simulink model "Modello_Irb1300_R2022a_ultima"  (R2022a)
settings: Solver=VariableStepAuto  StartTime=0.0  StopTime=37  RelTol=1e-3
undefined symbols (not defined in the file or in its folder): DiscIntNeverNeededParam
libraries: vrlib x3, simulink x1
settings Model: Creator=giaki  LastModifiedBy=adewa
settings ModelReferenceCC: EnableRefExpFcnMdlSchedulingChecks=off
settings RTWCC: Description=Generic Real-Time Target  GPUComputeCapability=5.0

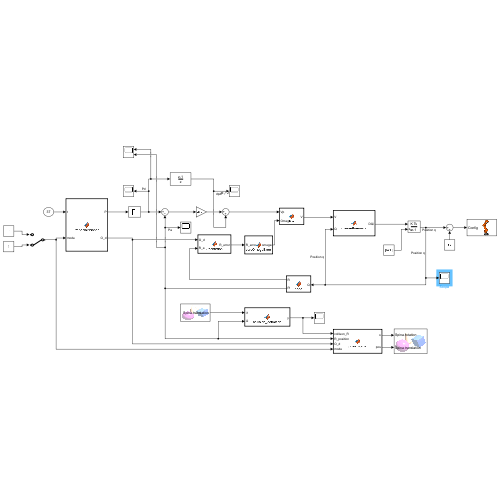
[thumbnail: Simulink's stored preview of the top-level diagram]
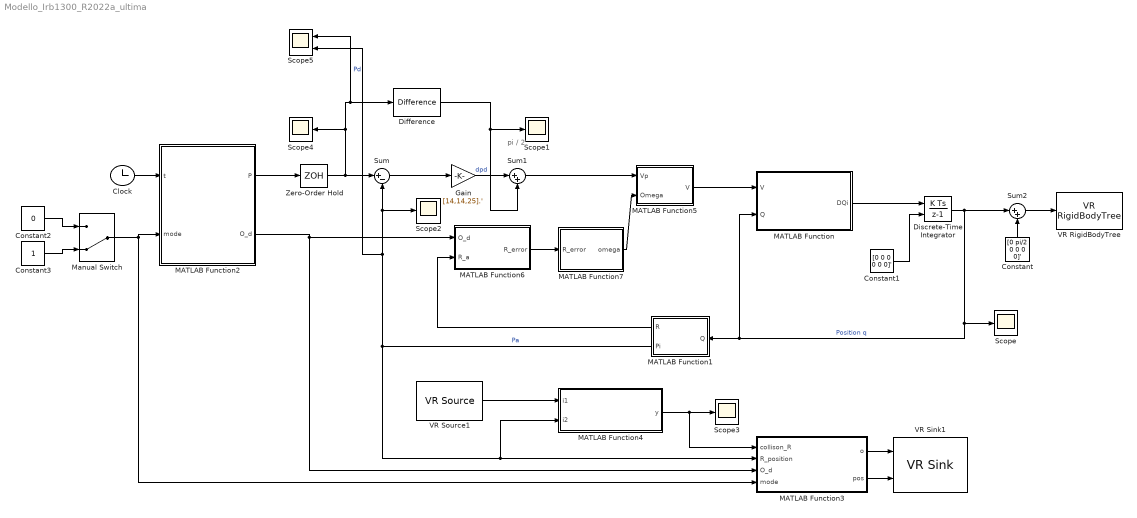
== system Modello_Irb1300_R2022a_ultima ==
  note: pi / 2
  Clock : Clock
  Constant : Constant  Value=[0 pi/2 0 0 0 0]'
  Constant1 : Constant  Value=[0 0 0 0 0 0]'
  Constant2 : Constant  Value=0
  Constant3 : Constant
  Difference : simulink/Discrete/Difference  ICPrevInput=[0.66, 0, 1.015].'  OutMin=[]  OutMax=[]  OutDataType=fixdt(1, 16)  OutScaling=2^-10  DoSatur=off
  Discrete-Time Integrator : DiscreteIntegrator  InitialConditionSource=external  SampleTime=-1  OutMin=[2]  ICPrevOutput=DiscIntNeverNeededParam  ICPrevScaledInput=DiscIntNeverNeededParam
  Gain : Gain  Gain=[14,14,25].'
  MATLAB Function : MATLAB Function  TreatAsAtomicUnit=on
  MATLAB Function1 : MATLAB Function  TreatAsAtomicUnit=on
  MATLAB Function2 : MATLAB Function  TreatAsAtomicUnit=on
  MATLAB Function3 : MATLAB Function  TreatAsAtomicUnit=on
  MATLAB Function4 : MATLAB Function  TreatAsAtomicUnit=on
  MATLAB Function5 : MATLAB Function  TreatAsAtomicUnit=on
  MATLAB Function6 : MATLAB Function  TreatAsAtomicUnit=on
  MATLAB Function7 : MATLAB Function  TreatAsAtomicUnit=on
  Manual Switch : ManualSwitch  CurrentSetting=0
  Scope{,1..4} (5 alike) : Scope
  Scope5 : Scope  NumInputPorts=2
  Sum : Sum  Inputs=|+-
  Sum1 : Sum  Inputs=|++
  Sum2 : Sum  Inputs=|++
  VR RigidBodyTree : vrlib/VR RigidBodyTree  VrmlFile=robot_scene_2.x3d  RBT=Irb1300  useRBT=on  Ts=0.1  ForceViewerOpen=on
      settings: SourceProductBaseCode=SL
  VR Sink1 : vrlib/VR Sink  InstantiateOnLoad=on  SampleTime=0.1  ViewEnable=on  RemoteChange=off  RemoteView=off  FieldsWritten=Spina.rotation.4.1.1.double#Spina.translation.3.1.1.double  WorldFileName=robot_scene_2.x3d  WorldDescription=Simple Robot Scene  AutoView=off  VideoDimensions=[]  AllowVariableSize=off
  VR Source1 : vrlib/VR Source  InstantiateOnLoad=on  SampleTime=0.1  ViewEnable=on  RemoteChange=off  RemoteView=off  FieldsRead=Spina.translation.1.3.1.double  WorldFileName=robot_scene_2.x3d  WorldDescription=Simple Robot Scene  AutoView=off  VideoDimensions=[]  AllowVariableSize=off
      settings: SourceProductBaseCode=SL
  Zero-Order Hold : ZeroOrderHold  SampleTime=0.05
  wires:
  Discrete-Time Integrator/1 -> Sum2/1, Scope/1, MATLAB Function/2(Q), MATLAB Function1/1(Q)  "Position q"
  Constant/1 -> Sum2/2
  Constant1/1 -> Discrete-Time Integrator/2
  Sum2/1 -> VR RigidBodyTree/1
  Difference/1 -> Scope1/1, Sum1/2  "dpd"
  Clock/1 -> MATLAB Function2/1(t)
  MATLAB Function/1(DQi) -> Discrete-Time Integrator/1
  Gain/1 -> Sum1/1
  MATLAB Function4/1(y) -> MATLAB Function3/1(collison_R), Scope3/1
  VR Source1/1 -> MATLAB Function4/1(i1)
  MATLAB Function2/1(P) -> Zero-Order Hold/1
  MATLAB Function3/2(pos) -> VR Sink1/2
  Zero-Order Hold/1 -> Scope4/1, Scope5/1, Difference/1, Sum/1  "Pd"
  Sum/1 -> Gain/1
  MATLAB Function1/1(R) -> MATLAB Function6/2(R_a)
  Sum1/1 -> MATLAB Function5/1(Vp)
  MATLAB Function5/1(V) -> MATLAB Function/1(V)
  MATLAB Function6/1(R_error) -> MATLAB Function7/1(R_error)
  MATLAB Function7/1(omega) -> MATLAB Function5/2(Omega)
  MATLAB Function1/2(Pi) -> Scope5/2, Sum/2, Scope2/1, MATLAB Function4/2(i2), MATLAB Function3/2(R_position)  "Pa"
  MATLAB Function2/2(O_d) -> MATLAB Function6/1(O_d), MATLAB Function3/3(O_d)
  MATLAB Function3/1(o) -> VR Sink1/1
  Manual Switch/1 -> MATLAB Function3/4(mode), MATLAB Function2/2(mode)
  Constant2/1 -> Manual Switch/1
  Constant3/1 -> Manual Switch/2

== matlab function Modello_Irb1300_R2022a_ultima/MATLAB Function1 ==
  data: R output; Q input; Pi output
function [R,Pi] = posa(Q)

th1 = Q(1);
th2 = Q(2);
th3 = Q(3);
th4 = Q(4);
th5 = Q(5);
th6 = Q(6);

% Matrice di trasformazione 4x4 calcolata nella posizione Q
T = [
    [sin(th6)*(cos(th4)*sin(th1) + sin(th4)*(cos(th1)*sin(th3)*sin(th2 + pi/2) - cos(th1)*cos(th3)*cos(th2 + pi/2))) + cos(th6)*(cos(th5)*(sin(th1)*sin(th4) - cos(th4)*(cos(th1)*sin(th3)*sin(th2 + pi/2) - cos(th1)*cos(th3)*cos(th2 + pi/2))) - sin(th5)*(cos(th1)*cos(th3)*sin(th2 + pi/2) + cos(th1)*cos(th2 + pi/2)*sin(th3))), cos(th6)*(cos(th4)*sin(th1) + sin(th4)*(cos(th1)*sin(th3)*sin(th2 + pi/2) - cos(th1)*cos(th3)*cos(th2 + pi/2))) - sin(th6)*(cos(th5)*(sin(th1)*sin(th4) - cos(th4)*(cos(th1)*sin(th3)*sin(th2 + pi/2) - cos(th1)*cos(th3)*cos(th2 + pi/2))) - sin(th5)*(cos(th1)*cos(th3)*sin(th2 + pi/2) + cos(th1)*cos(th2 + pi/2)*sin(th3))), sin(th5)*(sin(th1)*sin(th4) - cos(th4)*(cos(th1)*sin(th3)*sin(th2 + pi/2) - cos(th1)*cos(th3)*cos(th2 + pi/2))) + cos(th5)*(cos(th1)*cos(th3)*sin(th2 + pi/2) + cos(th1)*cos(th2 + pi/2)*sin(th3)), cos(th1)/20 + (17*cos(th1)*cos(th2 + pi/2))/40 + (9*sin(th5)*(sin(th1)*sin(th4) - cos(th4)*(cos(th1)*sin(th3)*sin(th2 + pi/2) - cos(th1)*cos(th3)*cos(th2 + pi/2))))/50 + (9*cos(th5)*(cos(th1)*cos(th3)*sin(th2 + pi/2) + cos(th1)*cos(th2 + pi/2)*sin(th3)))/50 + (17*cos(th1)*cos(th3)*sin(th2 + pi/2))/40 + (17*cos(th1)*cos(th2 + pi/2)*sin(th3))/40 - (cos(th1)*sin(th3)*sin(th2 + pi/2))/25 + (cos(th1)*cos(th3)*cos(th2 + pi/2))/25]
    [-sin(th6)*(cos(th1)*cos(th4) + sin(th4)*(cos(th3)*cos(th2 + pi/2)*sin(th1) - sin(th1)*sin(th3)*sin(th2 + pi/2))) - cos(th6)*(cos(th5)*(cos(th1)*sin(th4) - cos(th4)*(cos(th3)*cos(th2 + pi/2)*sin(th1) - sin(th1)*sin(th3)*sin(th2 + pi/2))) + sin(th5)*(cos(th3)*sin(th1)*sin(th2 + pi/2) + cos(th2 + pi/2)*sin(th1)*sin(th3))), sin(th6)*(cos(th5)*(cos(th1)*sin(th4) - cos(th4)*(cos(th3)*cos(th2 + pi/2)*sin(th1) - sin(th1)*sin(th3)*sin(th2 + pi/2))) + sin(th5)*(cos(th3)*sin(th1)*sin(th2 + pi/2) + cos(th2 + pi/2)*sin(th1)*sin(th3))) - cos(th6)*(cos(th1)*cos(th4) + sin(th4)*(cos(th3)*cos(th2 + pi/2)*sin(th1) - sin(th1)*sin(th3)*sin(th2 + pi/2))), cos(th5)*(cos(th3)*sin(th1)*sin(th2 + pi/2) + cos(th2 + pi/2)*sin(th1)*sin(th3)) - sin(th5)*(cos(th1)*sin(th4) - cos(th4)*(cos(th3)*cos(th2 + pi/2)*sin(th1) - sin(th1)*sin(th3)*sin(th2 + pi/2))), sin(th1)/20 + (17*cos(th2 + pi/2)*sin(th1))/40 - (9*sin(th5)*(cos(th1)*sin(th4) - cos(th4)*(cos(th3)*cos(th2 + pi/2)*sin(th1) - sin(th1)*sin(th3)*sin(th2 + pi/2))))/50 + (9*cos(th5)*(cos(th3)*sin(th1)*sin(th2 + pi/2) + cos(th2 + pi/2)*sin(th1)*sin(th3)))/50 + (cos(th3)*cos(th2 + pi/2)*sin(th1))/25 + (17*cos(th3)*sin(th1)*sin(th2 + pi/2))/40 + (17*cos(th2 + pi/2)*sin(th1)*sin(th3))/40 - (sin(th1)*sin(th3)*sin(th2 + pi/2))/25]
    [cos(th6)*(sin(th5)*(cos(th3)*cos(th2 + pi/2) - sin(th3)*sin(th2 + pi/2)) + cos(th4)*cos(th5)*(cos(th3)*sin(th2 + pi/2) + cos(th2 + pi/2)*sin(th3))) - sin(th4)*sin(th6)*(cos(th3)*sin(th2 + pi/2) + cos(th2 + pi/2)*sin(th3)), -sin(th6)*(sin(th5)*(cos(th3)*cos(th2 + pi/2) - sin(th3)*sin(th2 + pi/2)) + cos(th4)*cos(th5)*(cos(th3)*sin(th2 + pi/2) + cos(th2 + pi/2)*sin(th3))) - cos(th6)*sin(th4)*(cos(th3)*sin(th2 + pi/2) + cos(th2 + pi/2)*sin(th3)), cos(th4)*sin(th5)*(cos(th3)*sin(th2 + pi/2) + cos(th2 + pi/2)*sin(th3)) - cos(th5)*(cos(th3)*cos(th2 + pi/2) - sin(th3)*sin(th2 + pi/2)), (17*sin(th2 + pi/2))/40 - (17*cos(th3)*cos(th2 + pi/2))/40 + (cos(th3)*sin(th2 + pi/2))/25 + (cos(th2 + pi/2)*sin(th3))/25 + (17*sin(th3)*sin(th2 + pi/2))/40 - (9*cos(th5)*(cos(th3)*cos(th2 + pi/2) - sin(th3)*sin(th2 + pi/2)))/50 + (9*cos(th4)*sin(th5)*(cos(th3)*sin(th2 + pi/2) + cos(th2 + pi/2)*sin(th3)))/50 + 68/125]
    [0, 0, 0, 1]
];

% Estrai la posizione (3x1)
Pi_position = T(1:3, 4);

% Estrai la matrice di rotazione (3x3)
R = T(1:3, 1:3);


% Restituisci la posizione
Pi = [Pi_position];
end

== matlab function Modello_Irb1300_R2022a_ultima/MATLAB Function ==
  data: V input; DQi output; Q input
function DQi = inverseKinematic(V,Q)

th1 = Q(1);
th2 = Q(2);
th3 = Q(3);
th4 = Q(4);
th5 = Q(5);
th6 = Q(6);


% cosiderando sia le traslazioni che le orientazioni viene utilizzato il seguente J che si riferisce al jacobiano completo J = Jp + Jo 
J = [
[(9*sin(th5)*(cos(th1)*sin(th4) - cos(th4)*(cos(th3)*cos(th2 + pi/2)*sin(th1) - sin(th1)*sin(th3)*sin(th2 + pi/2))))/50 - (17*cos(th2 + pi/2)*sin(th1))/40 - sin(th1)/20 - (9*cos(th5)*(cos(th3)*sin(th1)*sin(th2 + pi/2) + cos(th2 + pi/2)*sin(th1)*sin(th3)))/50 - (cos(th3)*cos(th2 + pi/2)*sin(th1))/25 - (17*cos(th3)*sin(th1)*sin(th2 + pi/2))/40 - (17*cos(th2 + pi/2)*sin(th1)*sin(th3))/40 + (sin(th1)*sin(th3)*sin(th2 + pi/2))/25, (17*cos(th1)*cos(th3)*cos(th2 + pi/2))/40 - (9*cos(th5)*(cos(th1)*sin(th3)*sin(th2 + pi/2) - cos(th1)*cos(th3)*cos(th2 + pi/2)))/50 - (cos(th1)*cos(th3)*sin(th2 + pi/2))/25 - (cos(th1)*cos(th2 + pi/2)*sin(th3))/25 - (17*cos(th1)*sin(th3)*sin(th2 + pi/2))/40 - (9*cos(th4)*sin(th5)*(cos(th1)*cos(th3)*sin(th2 + pi/2) + cos(th1)*cos(th2 + pi/2)*sin(th3)))/50 - (17*cos(th1)*sin(th2 + pi/2))/40, (17*cos(th1)*cos(th3)*cos(th2 + pi/2))/40 - (cos(th1)*cos(th3)*sin(th2 + pi/2))/25 - (cos(th1)*cos(th2 + pi/2)*sin(th3))/25 - (17*cos(th1)*sin(th3)*sin(th2 + pi/2))/40 - (9*cos(th4)*sin(th5)*(cos(th1)*cos(th3)*sin(th2 + pi/2) + cos(th1)*cos(th2 + pi/2)*sin(th3)))/50 - (9*cos(th5)*(cos(th1)*sin(th3)*sin(th2 + pi/2) - cos(th1)*cos(th3)*cos(th2 + pi/2)))/50,  (9*sin(th5)*(cos(th4)*sin(th1) + sin(th4)*(cos(th1)*sin(th3)*sin(th2 + pi/2) - cos(th1)*cos(th3)*cos(th2 + pi/2))))/50,   (9*cos(th5)*(sin(th1)*sin(th4) - cos(th4)*(cos(th1)*sin(th3)*sin(th2 + pi/2) - cos(th1)*cos(th3)*cos(th2 + pi/2))))/50 - (9*sin(th5)*(cos(th1)*cos(th3)*sin(th2 + pi/2) + cos(th1)*cos(th2 + pi/2)*sin(th3)))/50,                                                                                                                                                                                                  0]
[cos(th1)/20 + (17*cos(th1)*cos(th2 + pi/2))/40 + (9*sin(th5)*(sin(th1)*sin(th4) - cos(th4)*(cos(th1)*sin(th3)*sin(th2 + pi/2) - cos(th1)*cos(th3)*cos(th2 + pi/2))))/50 + (9*cos(th5)*(cos(th1)*cos(th3)*sin(th2 + pi/2) + cos(th1)*cos(th2 + pi/2)*sin(th3)))/50 + (17*cos(th1)*cos(th3)*sin(th2 + pi/2))/40 + (17*cos(th1)*cos(th2 + pi/2)*sin(th3))/40 - (cos(th1)*sin(th3)*sin(th2 + pi/2))/25 + (cos(th1)*cos(th3)*cos(th2 + pi/2))/25, (9*cos(th5)*(cos(th3)*cos(th2 + pi/2)*sin(th1) - sin(th1)*sin(th3)*sin(th2 + pi/2)))/50 - (17*sin(th1)*sin(th2 + pi/2))/40 + (17*cos(th3)*cos(th2 + pi/2)*sin(th1))/40 - (cos(th3)*sin(th1)*sin(th2 + pi/2))/25 - (cos(th2 + pi/2)*sin(th1)*sin(th3))/25 - (17*sin(th1)*sin(th3)*sin(th2 + pi/2))/40 - (9*cos(th4)*sin(th5)*(cos(th3)*sin(th1)*sin(th2 + pi/2) + cos(th2 + pi/2)*sin(th1)*sin(th3)))/50, (9*cos(th5)*(cos(th3)*cos(th2 + pi/2)*sin(th1) - sin(th1)*sin(th3)*sin(th2 + pi/2)))/50 + (17*cos(th3)*cos(th2 + pi/2)*sin(th1))/40 - (cos(th3)*sin(th1)*sin(th2 + pi/2))/25 - (cos(th2 + pi/2)*sin(th1)*sin(th3))/25 - (17*sin(th1)*sin(th3)*sin(th2 + pi/2))/40 - (9*cos(th4)*sin(th5)*(cos(th3)*sin(th1)*sin(th2 + pi/2) + cos(th2 + pi/2)*sin(th1)*sin(th3)))/50, -(9*sin(th5)*(cos(th1)*cos(th4) + sin(th4)*(cos(th3)*cos(th2 + pi/2)*sin(th1) - sin(th1)*sin(th3)*sin(th2 + pi/2))))/50, - (9*cos(th5)*(cos(th1)*sin(th4) - cos(th4)*(cos(th3)*cos(th2 + pi/2)*sin(th1) - sin(th1)*sin(th3)*sin(th2 + pi/2))))/50 - (9*sin(th5)*(cos(th3)*sin(th1)*sin(th2 + pi/2) + cos(th2 + pi/2)*sin(th1)*sin(th3)))/50,                                                                                                                                                                                                  0]
[                                                                                                                                                                                                                                                                                                                                                                                                                                          0,                                                                                  (17*cos(th2 + pi/2))/40 + (cos(th3)*cos(th2 + pi/2))/25 + (17*cos(th3)*sin(th2 + pi/2))/40 + (17*cos(th2 + pi/2)*sin(th3))/40 - (sin(th3)*sin(th2 + pi/2))/25 + (9*cos(th5)*(cos(th3)*sin(th2 + pi/2) + cos(th2 + pi/2)*sin(th3)))/50 + (9*cos(th4)*sin(th5)*(cos(th3)*cos(th2 + pi/2) - sin(th3)*sin(th2 + pi/2)))/50,                                                                         (cos(th3)*cos(th2 + pi/2))/25 + (17*cos(th3)*sin(th2 + pi/2))/40 + (17*cos(th2 + pi/2)*sin(th3))/40 - (sin(th3)*sin(th2 + pi/2))/25 + (9*cos(th5)*(cos(th3)*sin(th2 + pi/2) + cos(th2 + pi/2)*sin(th3)))/50 + (9*cos(th4)*sin(th5)*(cos(th3)*cos(th2 + pi/2) - sin(th3)*sin(th2 + pi/2)))/50,                                         -(9*sin(th4)*sin(th5)*(cos(th3)*sin(th2 + pi/2) + cos(th2 + pi/2)*sin(th3)))/50,                                                             (9*sin(th5)*(cos(th3)*cos(th2 + pi/2) - sin(th3)*sin(th2 + pi/2)))/50 + (9*cos(th4)*cos(th5)*(cos(th3)*sin(th2 + pi/2) + cos(th2 + pi/2)*sin(th3)))/50,                                                                                                                                                                                                  0]
[                                                                                                                                                                                                                                                                                                                                                                                                                                          0,                                                                                                                                                                                                                                                                                                                                                                                                sin(th1),                                                                                                                                                                                                                                                                                                                                                             sin(th1),                                                   cos(th1)*cos(th3)*sin(th2 + pi/2) + cos(th1)*cos(th2 + pi/2)*sin(th3),                                                                                                               cos(th4)*sin(th1) + sin(th4)*(cos(th1)*sin(th3)*sin(th2 + pi/2) - cos(th1)*cos(th3)*cos(th2 + pi/2)), sin(th5)*(sin(th1)*sin(th4) - cos(th4)*(cos(th1)*sin(th3)*sin(th2 + pi/2) - cos(th1)*cos(th3)*cos(th2 + pi/2))) + cos(th5)*(cos(th1)*cos(th3)*sin(th2 + pi/2) + cos(th1)*cos(th2 + pi/2)*sin(th3))]
[                                                                                                                                                                                                                                                                                                                                                                                                                                          0,                                                                                                                                                                                                                                                                                                                                                                                               -cos(th1),                                                                                                                                                                                                                                                                                                                                                            -cos(th1),                                                   cos(th3)*sin(th1)*sin(th2 + pi/2) + cos(th2 + pi/2)*sin(th1)*sin(th3),                                                                                                             - cos(th1)*cos(th4) - sin(th4)*(cos(th3)*cos(th2 + pi/2)*sin(th1) - sin(th1)*sin(th3)*sin(th2 + pi/2)), cos(th5)*(cos(th3)*sin(th1)*sin(th2 + pi/2) + cos(th2 + pi/2)*sin(th1)*sin(th3)) - sin(th5)*(cos(th1)*sin(th4) - cos(th4)*(cos(th3)*cos(th2 + pi/2)*sin(th1) - sin(th1)*sin(th3)*sin(th2 + pi/2)))]
[                                                                                                                                                                                                                                                                                                                                                                                                                                          1,                                                                                                                                                                                                                                                                                                                                                                                                       0,                                                                                                                                                                                                                                                                                                                                                                    0,                                                                     sin(th3)*sin(th2 + pi/2) - cos(th3)*cos(th2 + pi/2),                                                                                                                                                    -sin(th4)*(cos(th3)*sin(th2 + pi/2) + cos(th2 + pi/2)*sin(th3)),                                                           cos(th4)*sin(th5)*(cos(th3)*sin(th2 + pi/2) + cos(th2 + pi/2)*sin(th3)) - cos(th5)*(cos(th3)*cos(th2 + pi/2) - sin(th3)*sin(th2 + pi/2))]
];


DQi = pinv(J)*V; % Matlab function for thr pseudo-inverse Matrix
pause (0.01);

end

== matlab function Modello_Irb1300_R2022a_ultima/MATLAB Function2 ==
  data: t input; P output; O_d output; mode input
function [P,O_d] = trapezioPlanner(t,mode)
    % Parametri per la traiettoria
    % Tempo di pianificazione
    % ogni tappa è definita come: 
    % struct('Pi', [Posizione inizale end effector], 'Pf', [posizione
    % finale end effector], 'tf', [durata della tappa], 'tw',[tempo di attesa a fine tappa],'O',[orientazione end effector]),
    %
    %struct('Pi', [X ; Y; Z], 'Pf', [X ; Y; Z], 'tf', [secondi], 'tw',[secondi],'O',[asse di rotazione X, asse di rotazione Y, asse di rotazione Z]),
    steps = [
            struct('Pi', [0.66; 1.015;   0], 'Pf', [0.55; 0.72; 0.45], 'tf', 15, 'tw', 5,'O',  [0, 0, 0]),        % Tappa 1
            struct('Pi', [0.55; 0.73; 0.45], 'Pf', [0.60; 0.70; 0.40], 'tf',  6, 'tw', 2,'O',  [0, 0, 0]),        % Tappa 2
            struct('Pi', [0.60; 0.70; 0.40], 'Pf', [0.55; 0.70; 0.40], 'tf',  6, 'tw', 2,'O',  [0, 0,-pi/2]),     % Tappa 3
            struct('Pi', [0.55; 0.70; 0.40], 'Pf', [0.55; 0.57; 0.14], 'tf', 15, 'tw', 5,'O',  [0, 0,-pi/2]),     % Tappa 4 
            struct('Pi', [0.55; 0.57; 0.14], 'Pf', [0.45; 0.57; 0.14], 'tf', 16, 'tw', 5,'O',  [0, 0,-pi/2])      % Tappa 4
            ];
    switch mode
        case 0
            steps = [
            struct('Pi', [0.66; 1.010;   0], 'Pf', [0.45; 0.72; 0.45], 'tf', 4, 'tw',  0.01,'O',  [0, 0, 0]),        % Tappa 1
            struct('Pi', [0.45; 0.70; 0.45], 'Pf', [0.60; 0.70; 0.40], 'tf', 4, 'tw',  0.01,'O',  [0, 0, 0]),        % Tappa 2
            struct('Pi', [0.60; 0.70; 0.40], 'Pf', [0.55; 0.70; 0.40], 'tf', 4, 'tw',  0.01,'O',  [0, 0,-pi/2]),     % Tappa 3
            struct('Pi', [0.55; 0.70; 0.40], 'Pf', [0.55; 0.57; 0.14], 'tf', 4, 'tw',  0.01,'O',  [0, 0,-pi/2]),     % Tappa 4 
            struct('Pi', [0.55; 0.57; 0.14], 'Pf', [0.45; 0.57; 0.14], 'tf', 4, 'tw',  0.01,'O',  [0, 0,-pi/2]),     % Tappa 5
            struct('Pi', [0.45; 0.57; 0.14], 'Pf', [0.66; 1.010;   0], 'tf', 6, 'tw', 14.95,'O',  [0, 0, 0])         % Tappa 6
            ];

        case 1
            steps = [
            struct('Pi', [0.66; 1.010;   0], 'Pf', [0.45; 0.57; 0.14], 'tf', 4, 'tw', 0.01,'O',   [0, 0, 0]),        % Tappa 1
            struct('Pi', [0.45; 0.57; 0.14], 'Pf', [0.55; 0.57; 0.14], 'tf', 4, 'tw', 0.01,'O',   [0, 0, -pi/2]),    % Tappa 2
            struct('Pi', [0.55; 0.57; 0.14], 'Pf', [0.55; 0.57; 0.20], 'tf', 4, 'tw', 0.01,'O',   [0, 0, -pi/2]),    % Tappa 3
            struct('Pi', [0.55; 0.57; 0.20], 'Pf', [0.55; 0.80; 0.40], 'tf', 4, 'tw', 0.01,'O',   [0, 0, -pi/2]),    % Tappa 4 
            struct('Pi', [0.55; 0.80; 0.40], 'Pf', [0.55; 0.70; 0.45], 'tf', 4, 'tw', 0.01,'O',   [0, 0, 0]),        % Tappa 5
            struct('Pi', [0.55; 0.70; 0.45], 'Pf', [0.45; 0.70; 0.45], 'tf', 4, 'tw', 0.01,'O',   [0, 0, 0]),        % Tappa 6
            struct('Pi', [0.45; 0.70; 0.45], 'Pf', [0.66; 1.010; 0],   'tf', 6, 'tw',  6.9,'O',   [0, 0, 0])          % Tappa 7
            ];
    end
    
   
    % Inizializzazione del tempo accumulato
    t_accum = 0; 
    
    % Matrice di trasformazione scena -> robot
    R_scene_to_robot = [ 1, 0,  0;   % x_s -> x_r
                         0, 0, -1;   % z_s -> -y_r
                         0, 1,  0];  % y_s -> z_r

    % Inizializzazione della posizione nello spazio scena
    
    P_scene = steps(1).Pi; % Posizione iniziale come fallback
    O_d = steps(1).O;      % orientazione iniziale come fallback
   
  % Calcolo della traiettoria lineare per ciascuna tappa
    for i = 1:length(steps)
        step = steps(i);
        
        % impostazione dell'orientazione dsiderata 
        O_d = step.O;

        % Tempo di inizio e fine della tappa
        t_start = t_accum;
        t_end = t_start + step.tf;
        
        % Controlla se il tempo attuale appartiene alla tappa corrente
        if t >= t_start && t < t_end
            % Calcola accelerazione
            delta_P = step.Pf - step.Pi;
            Acc = 4 * delta_P / step.tf^2; % Accelerazione necessaria

            % Calcola i tempi critici per il profilo trapezoidale
            sqrtTerm = sqrt(step.tf^2 / 4 - norm(delta_P) / norm(Acc));
            tc1 = step.tf / 2 - sqrtTerm;
            tc2 = step.tf / 2 + sqrtTerm;
            
            t_rel = t - t_start;

            % Calcolo posizione in base al profilo trapezoidale
            if t_rel >= 0 && t_rel < tc1
                % Fase di accelerazione
                P_scene = step.Pi + 1/2 * Acc * t_rel^2;
                
            elseif t_rel >= tc1 && t_rel < tc2
                % Fase a velocità costante
                P_scene = step.Pi + Acc * tc1 * (t_rel - tc1 / 2);
                
            elseif t_rel >= tc2 && t_rel < step.tf
                % Fase di decelerazione
                P_scene = step.Pf - 1/2 * Acc * (step.tf - t_rel)^2;
                
            end

            break; % Interrompe il loop dopo aver raggiunto la tappa corrente
        elseif t >= t_end && t < t_end + step.tw
            % Fase di attesa (mantiene la posizione finale della tappa)
            P_scene = step.Pf;
            break; % Interrompe il loop
        end

        % Aggiorna il tempo accumulato per la prossima tappa
        t_accum = t_end + step.tw;
    end
    
    % Conversione in coordinate robot
    position_robot = R_scene_to_robot * P_scene;
    % Uscita: combinazione di posizione, orientamento, velocità e accelerazioni
    P = [position_robot];
    %O_d = [theta,phi,psi];  % Rotazione attorno all'asse x 
    % Rotazione attorno all'asse y 
           
end

== matlab function Modello_Irb1300_R2022a_ultima/MATLAB Function3 ==
  data: collison_R input; R_position input; O_d input; mode input; o output; pos output
function [o,pos] = posa_spina(collison_R,R_position,O_d,mode)
     
     
     
     psi = O_d(3); % Rotazione attorno all'asse Z dell'end effector (Asse che punta verso il pezzo da agganciare)

     pos = [0.60; 0.7; 0.4];
     o = [0 0 0 0];

     
     
     % Viene utilizzata la matrice di rotazione R_robot_to_scene per
     % traformare la posizione del dell'end effector riferita alla terna
     % del robot R_position, in posizione dell'end effector riferita alla
     % scena
     R_robot_to_scene = [1,   0,   0;     
                         0,   0,   1;     
                         0,  -1,   0];
     
    robot_pos = R_robot_to_scene * R_position;
    
    %utilizziamo la variabile mode per individuare quale tipo Task abbiamo
    %simulando in questo modo possiamo impostare nel modo giusto la
    %posizione della spina 
    
    % Inizializzazione della variabile sgancio_spina di tipo persistente,
    % in questo modo è possibile tenere conto dello stato della variabile
    % in ogni istante mantenedo lo stato anche dopo il controllo

    persistent sgancio_spina;
    
     if isempty(sgancio_spina)
       sgancio_spina = 0;
    end
 

    if (mode == 0)   
        if (collison_R == 1)
            pos = robot_pos;
            if (psi == -pi/2)
                o = [1 0 0 -1.5708];
            end
        end
        if((abs(robot_pos(1) - 0.55) < 0.02) && (abs(robot_pos(2) - 0.57) < 0.02) && (abs(robot_pos(3) - 0.14) < 0.02))
            sgancio_spina = 1;
        end
        if(sgancio_spina == 1)
             pos = [0.55; 0.57; 0.14];
             o = [1 0 0 -1.5708];
        end

    elseif(mode == 1)

        pos = [0.55; 0.57; 0.14];
        o = [1 0 0 -1.5708];
        if (collison_R == 1)
            pos = robot_pos;
            if (psi == -pi/2)
                o = [1 0 0 -1.5708];
            elseif (psi == 0)
                 o = [1 0 0 0];
            end
            
        end

        if((abs(robot_pos(1) - 0.55) < 0.005) && (abs(robot_pos(2) - 0.70) < 0.005) && (abs(robot_pos(3) - 0.45) < 0.005))
            sgancio_spina = 1;
        end

        if(sgancio_spina == 1)
             pos = [0.55; 0.70; 0.45];
             o = [1 0 0 0];
        end
    end
end

== matlab function Modello_Irb1300_R2022a_ultima/MATLAB Function4 ==
  data: i1 input; y output; i2 input
function y  = collision_detection(i1, i2)
   % Trasformazione dal frame della scena al frame del robot
   R_scene_to_robot = [1,  0,  0;     % x_s -> x_r
                       0,  0, -1;     % z_s -> -y_r
                       0, 1,   0];    % y_s -> z_r

   % Applicazione della trasformazione a i1
   i1_robot = R_scene_to_robot * i1;

   % Coordinate di i1 nel frame del robot

   xi1 = i1_robot(1); % Asse X del robot
   yi1 = i1_robot(2); % Asse Y del robot
   zi1 = i1_robot(3); % Asse Z del robot

   % Coordinate di i2 nel frame del robot
   xi2 = i2(1,1);
   yi2 = i2(2,1);
   zi2 = i2(3,1);

   % Inizializzazione del risultato
   y = 0;

   % Controllo collisione
   if ((abs(xi1 - xi2) < 0.02) && (abs(yi1 - yi2) < 0.02) && (abs(zi1 - zi2) < 0.02))
       y = 1;
   end
end

== matlab function Modello_Irb1300_R2022a_ultima/MATLAB Function5 ==
  data: Vp input; V output; Omega input
function V = fcn(Vp,Omega)
% Questa funzione a partire dalle velocità delle Velocità Vp e le
% orientazioni creo il vettore V [6x1]
V = [Vp;Omega];

== matlab function Modello_Irb1300_R2022a_ultima/MATLAB Function6 ==
  data: O_d input; R_error output; R_a input
function R_error = Orientation(O_d,R_a)
% R_a, è la matrice di rotazione ottenuta dalla posa in retroazione 

%R_iniziale, questa matrice è la matrice iniziale (orientazione assoluta) 
%che permette di riferire gli angoli di eulero alla orientazione relativa dell'end effector

R_iniziale = [
    0.0000    0.0000    1.0000 ;
    1.0000         0    0.0000 ;
         0    1.0000    0.0000 ];

% Angoli pi di Eulero in radianti
theta = O_d(1);          % Rotazione attorno all'asse x 
  phi = O_d(2);          % Rotazione attorno all'asse y 
  psi = O_d(3) + pi/2 ;  % Rotazione attorno all'asse z (per corretta posizione a riposo)

% Matrici di rotazione elementari
R_x = [
      1, 0, 0;
      0, cos(theta), -sin(theta);
      0, sin(theta), cos(theta)
];

R_y = [
    cos(phi), 0, sin(phi);
    0, 1, 0;
    -sin(phi), 0, cos(phi)
];

R_z = [
    cos(psi), -sin(psi), 0;
    sin(psi), cos(psi), 0;
    0, 0, 1
];

% Matrice di rotazione totale
% R_d_rel consiste nella matrice di Rotazione Desiderate relativa all'endeffector
R_d_rel = R_z * R_y * R_x;  % Ordine: ZYX (dipende dalla convenzione scelta)

%R_d_ass consiste nella matrice di rotazione desiderata assoluta espressa
%rispetto la terna di base del robot 
R_d_ass = R_iniziale * R_d_rel;

% Calcolo del'errore angolare R_error
% Prodotto della matrice di rotazione desderata per la trasposta
% della matrice di Rotazione attuale 
R_error = R_d_ass * R_a';

end

== matlab function Modello_Irb1300_R2022a_ultima/MATLAB Function7 ==
  data: R_error input; omega output
 function omega = calcOmegaError(R_error)
    % Calcola la matrice di errore

    % Calcola theta
    theta = acos((trace(R_error) - 1) / 2);

    % Calcola matrice antisimmetrica u_hat
    if abs(theta) < 1e-6  % Evita divisioni per zero
        omega = [0;0;0];
    else
        skew_matrix = (R_error - R_error')/(2*sin(theta));  % Caso limite (errore molto piccolo)
        omega = [skew_matrix(3,2);skew_matrix(1,3);skew_matrix(2,1)];
    end

    % Estrai omega_e usando vex
    omega = theta * omega;
end
